simulink model "HighController"  (R2023a)
settings: Solver=VariableStepAuto  StartTime=0.0  StopTime=10.0  RelTol=1e-3
settings Model: Creator=lehas  LastModifiedBy=lehas

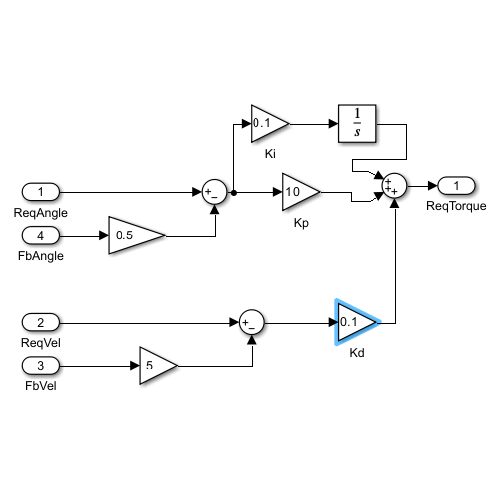
[thumbnail: Simulink's stored preview of the top-level diagram]
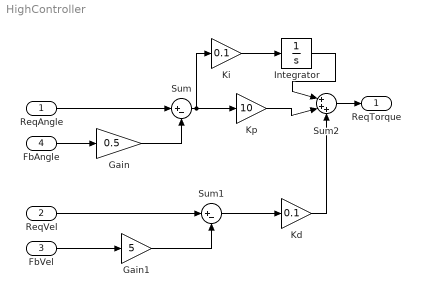
== system HighController ==
  ReqAngle : Inport
  ReqVel : Inport  Port=2
  FbVel : Inport  Port=3
  FbAngle : Inport  Port=4
  Gain : Gain  Gain=0.5
  Gain1 : Gain  Gain=5
  Integrator : Integrator
  Kd : Gain  Gain=0.1
  Ki : Gain  Gain=0.1
  Kp : Gain  Gain=10
  Sum : Sum  Inputs=|+-
  Sum1 : Sum  Inputs=|+-
  Sum2 : Sum  Inputs=|+++
  ReqTorque : Outport
  wires:
  FbAngle/1 -> Gain/1
  ReqAngle/1 -> Sum/1
  Gain/1 -> Sum/2
  FbVel/1 -> Gain1/1
  ReqVel/1 -> Sum1/1
  Gain1/1 -> Sum1/2
  Ki/1 -> Integrator/1
  Integrator/1 -> Sum2/1
  Sum/1 -> Ki/1, Kp/1
  Kp/1 -> Sum2/2
  Sum1/1 -> Kd/1
  Kd/1 -> Sum2/3
  Sum2/1 -> ReqTorque/1
